simulink model "secondpathEstimator"  (R2020b)
settings: Solver=VariableStepAuto  StartTime=0.0  StopTime=10  RelTol=1e-3
libraries: dspsrcs4 x1, dspadpt3 x1
settings Model: Creator=Borma  LastModifiedBy=Borma

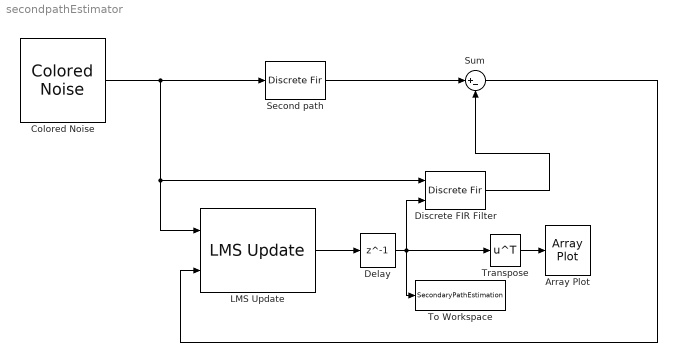
== system secondpathEstimator ==
  Array Plot : ArrayPlot
  Colored Noise : dspsrcs4/Colored Noise  Color=white  InverseFrequencyPower=1  BoundedOutput=off  NumChannels=1  OutputDataType=double  SamplesPerFrame=1  SampleTime=1/4000  RandomStream=mt19937ar with seed  Seed=67  SimulateUsing=Interpreted execution
      settings: SourceProductBaseCode=DS
  Delay : Delay  DelayLength=1  InitialCondition=0
  Discrete FIR Filter : DiscreteFir  CoefSource=Input port  InputProcessing=Columns as channels (frame based)
      settings: InputPortMap=u0,u1
  LMS Update : dspadpt3/LMS Update  Method=Normalized LMS  Length=24  StepSizeSource=Property  StepSize=0.01  LeakageFactor=1.0  InitialConditions=0  EnableAdaptInput=off  EnableResetInput=off  SimulateUsing=Code generation
      settings: SourceProductBaseCode=DS
  Second path : DiscreteFir  Coefficients=[0 0 -0.5 -0.5 -0.3 0.2 -0.1 0.5 -0.5]
  Sum : Sum  Inputs=|+-
  To Workspace : ToWorkspace  VariableName=SecondaryPathEstimation  SampleTime=1
      settings: Save2DSignal=2-D array (concatenate along first dimension)
  Transpose : Math  Operator=transpose  SaturateOnIntegerOverflow=on
  wires:
  Colored Noise/1 -> Second path/1, Discrete FIR Filter/1, LMS Update/1
  Second path/1 -> Sum/1
  Sum/1 -> LMS Update/2
  LMS Update/1 -> Delay/1
  Delay/1 -> To Workspace/1, Discrete FIR Filter/2, Transpose/1
  Transpose/1 -> Array Plot/1
  Discrete FIR Filter/1 -> Sum/2
